simulink model "Ex_1_4_Control_Puma_2019a"  (R2019a)
settings: Solver=FixedStepAuto  StartTime=0.0  StopTime=6  FixedStep=0.01  RelTol=1e-3
libraries: simulink x6
(part 1 of 2)
settings Model: Creator=s3818101  LastModifiedBy=s3818101
settings DebuggingCC: UnconnectedInputMsg=none  UnconnectedOutputMsg=none  UnconnectedLineMsg=none
settings ModelReferenceCC: EnableRefExpFcnMdlSchedulingChecks=off
settings RTWCC: Description=Generic Real-Time Target

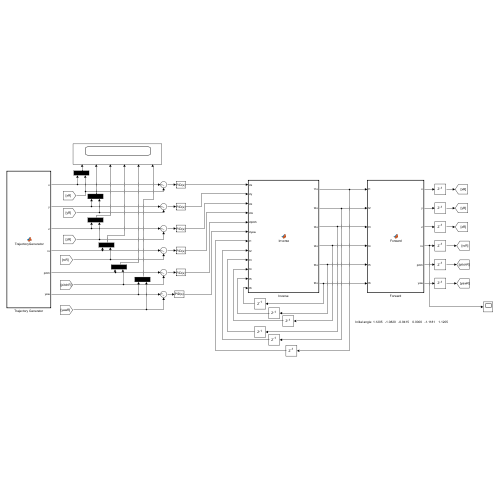
[thumbnail: Simulink's stored preview of the top-level diagram]
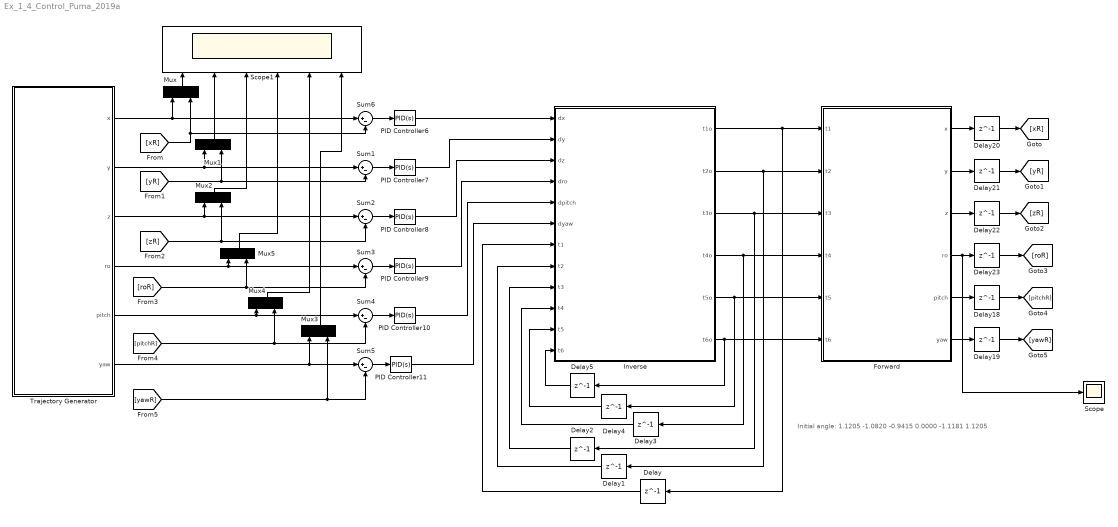
== system Ex_1_4_Control_Puma_2019a ==
  note: Initial angle: 1.1205 -1.0820 -0.9415 0.0000 -1.1181 1.1205
  Delay : Delay  DelayLength=1  InitialCondition=1.1205
  Delay1 : Delay  DelayLength=1  InitialCondition=-1.1181
  Delay18 : Delay  DelayLength=1  InitialCondition=0
  Delay19 : Delay  DelayLength=1  InitialCondition=0
  Delay2 : Delay  DelayLength=1  InitialCondition=0.001
  Delay20 : Delay  DelayLength=1  InitialCondition=0.001
  Delay21 : Delay  DelayLength=1  InitialCondition=0.001
  Delay22 : Delay  DelayLength=1  InitialCondition=0.01
  Delay23 : Delay  DelayLength=1  InitialCondition=pi
  Delay3 : Delay  DelayLength=1  InitialCondition=-0.9415
  Delay4 : Delay  DelayLength=1  InitialCondition=-1.082
  Delay5 : Delay  DelayLength=1  InitialCondition=1.1205
  "Forward " : MATLAB Function  TreatAsAtomicUnit=on
  Inverse : MATLAB Function  TreatAsAtomicUnit=on
  Mux{,1..5} (6 alike) : Mux  Inputs=2
  PID Controller10 : simulink/Continuous/PID Controller  Controller=PID  Form=Parallel  TimeDomain=Continuous-time  SampleTime=-1  IntegratorMethod=Forward Euler  ControllerParametersSource=internal  P=3.6  I=0  D=0.1  N=100  UseFilter=on  TunerSelectOption=Transfer Function Based (PID Tuner App)  InitialConditionSource=internal  InitialConditionForIntegrator=0  InitialConditionForFilter=0  DifferentiatorICPrevScaledInput=0  ExternalReset=none  TrackingMode=off  Kt=1  LimitOutput=off  UpperSaturationLimit=inf  LowerSaturationLimit=-inf  LinearizeAsGain=on  AntiWindupMode=none  Kb=1  POutMin=[]  POutMax=[]  IOutMin=[]  IOutMax=[]  DOutMin=[]  DOutMax=[]  NOutMin=[]  NOutMax=[]  SumOutMin=[]  SumOutMax=[]  SaturationOutMin=[]  SaturationOutMax=[]  PParamMin=[]  PParamMax=[]  IParamMin=[]  IParamMax=[]  DParamMin=[]  DParamMax=[]  NParamMin=[]  NParamMax=[]  KbParamMin=[]  KbParamMax=[]  KtParamMin=[]  KtParamMax=[]  KbOutMin=[]  KbOutMax=[]  KtOutMin=[]  KtOutMax=[]  IntegratorOutMin=[]  IntegratorOutMax=[]  FilterOutMin=[]  FilterOutMax=[]  SumI1OutMin=[]  SumI1OutMax=[]  SumI2OutMin=[]  SumI2OutMax=[]  SumI3OutMin=[]  SumI3OutMax=[]  SumI4OutMin=[]  SumI4OutMax=[]  SumDOutMin=[]  SumDOutMax=[]  DifferentiatorOutMin=[]  DifferentiatorOutMax=[]  FilterDiffOutCoefMin=[]  FilterDiffOutCoefMax=[]  ReciprocalOutMin=[]  ReciprocalOutMax=[]  SumDenOutMin=[]  SumDenOutMax=[]  SumNumOutMin=[]  SumNumOutMax=[]  DivideOutMin=[]  DivideOutMax=[]  IntegratorContinuousStateAttributes=''  IntegratorStateMustResolveToSignalObject=off  IntegratorRTWStateStorageClass=Auto  FilterContinuousStateAttributes=''  FilterStateMustResolveToSignalObject=off  FilterRTWStateStorageClass=Auto  ParallelPVariant=InternalParameters  IdealPVariant=Disabled  IVariant=InternalParameters  DVariant=InternalParameters  IntegratorVariant=Continuous  SatVariant=Disabled  AWVariant=Passthrough  PCopyVariant=Disabled  TRVariant=Disabled  FdbkBlocksVariant=Forward  IdealPFdbkVariant=Disabled  SatFdbkVariant=Disabled  DerivativeFilterVariant=ContFilter  NVariant=InternalParameters  NCopyVariant=Disabled  FilterICVariant=InternalICsFilter  IntegratorICVariant=InternalICs  ExternalResetVariant=Disabled  TRSumVariant=Passthrough  SumFdbkVariant=Disabled  SumVariant=Sum_PID
  PID Controller11 : simulink/Continuous/PID Controller  Controller=PID  Form=Parallel  TimeDomain=Continuous-time  SampleTime=-1  IntegratorMethod=Forward Euler  ControllerParametersSource=internal  P=3  I=0  D=0.008  N=100  UseFilter=on  TunerSelectOption=Transfer Function Based (PID Tuner App)  InitialConditionSource=internal  InitialConditionForIntegrator=0  InitialConditionForFilter=0  DifferentiatorICPrevScaledInput=0  ExternalReset=none  TrackingMode=off  Kt=1  LimitOutput=off  UpperSaturationLimit=inf  LowerSaturationLimit=-inf  LinearizeAsGain=on  AntiWindupMode=none  Kb=1  POutMin=[]  POutMax=[]  IOutMin=[]  IOutMax=[]  DOutMin=[]  DOutMax=[]  NOutMin=[]  NOutMax=[]  SumOutMin=[]  SumOutMax=[]  SaturationOutMin=[]  SaturationOutMax=[]  PParamMin=[]  PParamMax=[]  IParamMin=[]  IParamMax=[]  DParamMin=[]  DParamMax=[]  NParamMin=[]  NParamMax=[]  KbParamMin=[]  KbParamMax=[]  KtParamMin=[]  KtParamMax=[]  KbOutMin=[]  KbOutMax=[]  KtOutMin=[]  KtOutMax=[]  IntegratorOutMin=[]  IntegratorOutMax=[]  FilterOutMin=[]  FilterOutMax=[]  SumI1OutMin=[]  SumI1OutMax=[]  SumI2OutMin=[]  SumI2OutMax=[]  SumI3OutMin=[]  SumI3OutMax=[]  SumI4OutMin=[]  SumI4OutMax=[]  SumDOutMin=[]  SumDOutMax=[]  DifferentiatorOutMin=[]  DifferentiatorOutMax=[]  FilterDiffOutCoefMin=[]  FilterDiffOutCoefMax=[]  ReciprocalOutMin=[]  ReciprocalOutMax=[]  SumDenOutMin=[]  SumDenOutMax=[]  SumNumOutMin=[]  SumNumOutMax=[]  DivideOutMin=[]  DivideOutMax=[]  IntegratorContinuousStateAttributes=''  IntegratorStateMustResolveToSignalObject=off  IntegratorRTWStateStorageClass=Auto  FilterContinuousStateAttributes=''  FilterStateMustResolveToSignalObject=off  FilterRTWStateStorageClass=Auto  ParallelPVariant=InternalParameters  IdealPVariant=Disabled  IVariant=InternalParameters  DVariant=InternalParameters  IntegratorVariant=Continuous  SatVariant=Disabled  AWVariant=Passthrough  PCopyVariant=Disabled  TRVariant=Disabled  FdbkBlocksVariant=Forward  IdealPFdbkVariant=Disabled  SatFdbkVariant=Disabled  DerivativeFilterVariant=ContFilter  NVariant=InternalParameters  NCopyVariant=Disabled  FilterICVariant=InternalICsFilter  IntegratorICVariant=InternalICs  ExternalResetVariant=Disabled  TRSumVariant=Passthrough  SumFdbkVariant=Disabled  SumVariant=Sum_PID
  PID Controller6 : simulink/Continuous/PID Controller  Controller=PID  Form=Parallel  TimeDomain=Continuous-time  SampleTime=-1  IntegratorMethod=Forward Euler  ControllerParametersSource=internal  P=10  I=0  D=0  N=100  UseFilter=on  TunerSelectOption=Transfer Function Based (PID Tuner App)  InitialConditionSource=internal  InitialConditionForIntegrator=0  InitialConditionForFilter=0  DifferentiatorICPrevScaledInput=0  ExternalReset=none  TrackingMode=off  Kt=1  LimitOutput=off  UpperSaturationLimit=inf  LowerSaturationLimit=-inf  LinearizeAsGain=on  AntiWindupMode=none  Kb=1  POutMin=[]  POutMax=[]  IOutMin=[]  IOutMax=[]  DOutMin=[]  DOutMax=[]  NOutMin=[]  NOutMax=[]  SumOutMin=[]  SumOutMax=[]  SaturationOutMin=[]  SaturationOutMax=[]  PParamMin=[]  PParamMax=[]  IParamMin=[]  IParamMax=[]  DParamMin=[]  DParamMax=[]  NParamMin=[]  NParamMax=[]  KbParamMin=[]  KbParamMax=[]  KtParamMin=[]  KtParamMax=[]  KbOutMin=[]  KbOutMax=[]  KtOutMin=[]  KtOutMax=[]  IntegratorOutMin=[]  IntegratorOutMax=[]  FilterOutMin=[]  FilterOutMax=[]  SumI1OutMin=[]  SumI1OutMax=[]  SumI2OutMin=[]  SumI2OutMax=[]  SumI3OutMin=[]  SumI3OutMax=[]  SumI4OutMin=[]  SumI4OutMax=[]  SumDOutMin=[]  SumDOutMax=[]  DifferentiatorOutMin=[]  DifferentiatorOutMax=[]  FilterDiffOutCoefMin=[]  FilterDiffOutCoefMax=[]  ReciprocalOutMin=[]  ReciprocalOutMax=[]  SumDenOutMin=[]  SumDenOutMax=[]  SumNumOutMin=[]  SumNumOutMax=[]  DivideOutMin=[]  DivideOutMax=[]  IntegratorContinuousStateAttributes=''  IntegratorStateMustResolveToSignalObject=off  IntegratorRTWStateStorageClass=Auto  FilterContinuousStateAttributes=''  FilterStateMustResolveToSignalObject=off  FilterRTWStateStorageClass=Auto  ParallelPVariant=InternalParameters  IdealPVariant=Disabled  IVariant=InternalParameters  DVariant=InternalParameters  IntegratorVariant=Continuous  SatVariant=Disabled  AWVariant=Passthrough  PCopyVariant=Disabled  TRVariant=Disabled  FdbkBlocksVariant=Forward  IdealPFdbkVariant=Disabled  SatFdbkVariant=Disabled  DerivativeFilterVariant=ContFilter  NVariant=InternalParameters  NCopyVariant=Disabled  FilterICVariant=InternalICsFilter  IntegratorICVariant=InternalICs  ExternalResetVariant=Disabled  TRSumVariant=Passthrough  SumFdbkVariant=Disabled  SumVariant=Sum_PID
  PID Controller7 : simulink/Continuous/PID Controller  Controller=PID  Form=Parallel  TimeDomain=Continuous-time  SampleTime=-1  IntegratorMethod=Forward Euler  ControllerParametersSource=internal  P=6  I=0  D=0  N=100  UseFilter=on  TunerSelectOption=Transfer Function Based (PID Tuner App)  InitialConditionSource=internal  InitialConditionForIntegrator=0  InitialConditionForFilter=0  DifferentiatorICPrevScaledInput=0  ExternalReset=none  TrackingMode=off  Kt=1  LimitOutput=off  UpperSaturationLimit=inf  LowerSaturationLimit=-inf  LinearizeAsGain=on  AntiWindupMode=none  Kb=1  POutMin=[]  POutMax=[]  IOutMin=[]  IOutMax=[]  DOutMin=[]  DOutMax=[]  NOutMin=[]  NOutMax=[]  SumOutMin=[]  SumOutMax=[]  SaturationOutMin=[]  SaturationOutMax=[]  PParamMin=[]  PParamMax=[]  IParamMin=[]  IParamMax=[]  DParamMin=[]  DParamMax=[]  NParamMin=[]  NParamMax=[]  KbParamMin=[]  KbParamMax=[]  KtParamMin=[]  KtParamMax=[]  KbOutMin=[]  KbOutMax=[]  KtOutMin=[]  KtOutMax=[]  IntegratorOutMin=[]  IntegratorOutMax=[]  FilterOutMin=[]  FilterOutMax=[]  SumI1OutMin=[]  SumI1OutMax=[]  SumI2OutMin=[]  SumI2OutMax=[]  SumI3OutMin=[]  SumI3OutMax=[]  SumI4OutMin=[]  SumI4OutMax=[]  SumDOutMin=[]  SumDOutMax=[]  DifferentiatorOutMin=[]  DifferentiatorOutMax=[]  FilterDiffOutCoefMin=[]  FilterDiffOutCoefMax=[]  ReciprocalOutMin=[]  ReciprocalOutMax=[]  SumDenOutMin=[]  SumDenOutMax=[]  SumNumOutMin=[]  SumNumOutMax=[]  DivideOutMin=[]  DivideOutMax=[]  IntegratorContinuousStateAttributes=''  IntegratorStateMustResolveToSignalObject=off  IntegratorRTWStateStorageClass=Auto  FilterContinuousStateAttributes=''  FilterStateMustResolveToSignalObject=off  FilterRTWStateStorageClass=Auto  ParallelPVariant=InternalParameters  IdealPVariant=Disabled  IVariant=InternalParameters  DVariant=InternalParameters  IntegratorVariant=Continuous  SatVariant=Disabled  AWVariant=Passthrough  PCopyVariant=Disabled  TRVariant=Disabled  FdbkBlocksVariant=Forward  IdealPFdbkVariant=Disabled  SatFdbkVariant=Disabled  DerivativeFilterVariant=ContFilter  NVariant=InternalParameters  NCopyVariant=Disabled  FilterICVariant=InternalICsFilter  IntegratorICVariant=InternalICs  ExternalResetVariant=Disabled  TRSumVariant=Passthrough  SumFdbkVariant=Disabled  SumVariant=Sum_PID
  PID Controller8 : simulink/Continuous/PID Controller  Controller=PID  Form=Parallel  TimeDomain=Continuous-time  SampleTime=-1  IntegratorMethod=Forward Euler  ControllerParametersSource=internal  P=6  I=0  D=0  N=100  UseFilter=on  TunerSelectOption=Transfer Function Based (PID Tuner App)  InitialConditionSource=internal  InitialConditionForIntegrator=0  InitialConditionForFilter=0  DifferentiatorICPrevScaledInput=0  ExternalReset=none  TrackingMode=off  Kt=1  LimitOutput=off  UpperSaturationLimit=inf  LowerSaturationLimit=-inf  LinearizeAsGain=on  AntiWindupMode=none  Kb=1  POutMin=[]  POutMax=[]  IOutMin=[]  IOutMax=[]  DOutMin=[]  DOutMax=[]  NOutMin=[]  NOutMax=[]  SumOutMin=[]  SumOutMax=[]  SaturationOutMin=[]  SaturationOutMax=[]  PParamMin=[]  PParamMax=[]  IParamMin=[]  IParamMax=[]  DParamMin=[]  DParamMax=[]  NParamMin=[]  NParamMax=[]  KbParamMin=[]  KbParamMax=[]  KtParamMin=[]  KtParamMax=[]  KbOutMin=[]  KbOutMax=[]  KtOutMin=[]  KtOutMax=[]  IntegratorOutMin=[]  IntegratorOutMax=[]  FilterOutMin=[]  FilterOutMax=[]  SumI1OutMin=[]  SumI1OutMax=[]  SumI2OutMin=[]  SumI2OutMax=[]  SumI3OutMin=[]  SumI3OutMax=[]  SumI4OutMin=[]  SumI4OutMax=[]  SumDOutMin=[]  SumDOutMax=[]  DifferentiatorOutMin=[]  DifferentiatorOutMax=[]  FilterDiffOutCoefMin=[]  FilterDiffOutCoefMax=[]  ReciprocalOutMin=[]  ReciprocalOutMax=[]  SumDenOutMin=[]  SumDenOutMax=[]  SumNumOutMin=[]  SumNumOutMax=[]  DivideOutMin=[]  DivideOutMax=[]  IntegratorContinuousStateAttributes=''  IntegratorStateMustResolveToSignalObject=off  IntegratorRTWStateStorageClass=Auto  FilterContinuousStateAttributes=''  FilterStateMustResolveToSignalObject=off  FilterRTWStateStorageClass=Auto  ParallelPVariant=InternalParameters  IdealPVariant=Disabled  IVariant=InternalParameters  DVariant=InternalParameters  IntegratorVariant=Continuous  SatVariant=Disabled  AWVariant=Passthrough  PCopyVariant=Disabled  TRVariant=Disabled  FdbkBlocksVariant=Forward  IdealPFdbkVariant=Disabled  SatFdbkVariant=Disabled  DerivativeFilterVariant=ContFilter  NVariant=InternalParameters  NCopyVariant=Disabled  FilterICVariant=InternalICsFilter  IntegratorICVariant=InternalICs  ExternalResetVariant=Disabled  TRSumVariant=Passthrough  SumFdbkVariant=Disabled  SumVariant=Sum_PID
  PID Controller9 : simulink/Continuous/PID Controller  Controller=PID  Form=Parallel  TimeDomain=Continuous-time  SampleTime=-1  IntegratorMethod=Forward Euler  ControllerParametersSource=internal  P=1  I=0  D=0.01  N=100  UseFilter=on  TunerSelectOption=Transfer Function Based (PID Tuner App)  InitialConditionSource=internal  InitialConditionForIntegrator=0  InitialConditionForFilter=0  DifferentiatorICPrevScaledInput=0  ExternalReset=none  TrackingMode=off  Kt=1  LimitOutput=off  UpperSaturationLimit=inf  LowerSaturationLimit=-inf  LinearizeAsGain=on  AntiWindupMode=none  Kb=1  POutMin=[]  POutMax=[]  IOutMin=[]  IOutMax=[]  DOutMin=[]  DOutMax=[]  NOutMin=[]  NOutMax=[]  SumOutMin=[]  SumOutMax=[]  SaturationOutMin=[]  SaturationOutMax=[]  PParamMin=[]  PParamMax=[]  IParamMin=[]  IParamMax=[]  DParamMin=[]  DParamMax=[]  NParamMin=[]  NParamMax=[]  KbParamMin=[]  KbParamMax=[]  KtParamMin=[]  KtParamMax=[]  KbOutMin=[]  KbOutMax=[]  KtOutMin=[]  KtOutMax=[]  IntegratorOutMin=[]  IntegratorOutMax=[]  FilterOutMin=[]  FilterOutMax=[]  SumI1OutMin=[]  SumI1OutMax=[]  SumI2OutMin=[]  SumI2OutMax=[]  SumI3OutMin=[]  SumI3OutMax=[]  SumI4OutMin=[]  SumI4OutMax=[]  SumDOutMin=[]  SumDOutMax=[]  DifferentiatorOutMin=[]  DifferentiatorOutMax=[]  FilterDiffOutCoefMin=[]  FilterDiffOutCoefMax=[]  ReciprocalOutMin=[]  ReciprocalOutMax=[]  SumDenOutMin=[]  SumDenOutMax=[]  SumNumOutMin=[]  SumNumOutMax=[]  DivideOutMin=[]  DivideOutMax=[]  IntegratorContinuousStateAttributes=''  IntegratorStateMustResolveToSignalObject=off  IntegratorRTWStateStorageClass=Auto  FilterContinuousStateAttributes=''  FilterStateMustResolveToSignalObject=off  FilterRTWStateStorageClass=Auto  ParallelPVariant=InternalParameters  IdealPVariant=Disabled  IVariant=InternalParameters  DVariant=InternalParameters  IntegratorVariant=Continuous  SatVariant=Disabled  AWVariant=Passthrough  PCopyVariant=Disabled  TRVariant=Disabled  FdbkBlocksVariant=Forward  IdealPFdbkVariant=Disabled  SatFdbkVariant=Disabled  DerivativeFilterVariant=ContFilter  NVariant=InternalParameters  NCopyVariant=Disabled  FilterICVariant=InternalICsFilter  IntegratorICVariant=InternalICs  ExternalResetVariant=Disabled  TRSumVariant=Passthrough  SumFdbkVariant=Disabled  SumVariant=Sum_PID
  Scope : Scope
  Scope1 : Scope  NumInputPorts=6
  Sum{1..6} (6 alike) : Sum  Inputs=|+-
  Trajectory Generator : MATLAB Function  TreatAsAtomicUnit=on
  wires:
  Trajectory Generator/1(x) -> Sum6/1, Mux/1
  "Forward "/1(x) -> Delay20/1
  "Forward "/2(y) -> Delay21/1
  "Forward "/3(z) -> Delay22/1
  Inverse/1(t1o) -> Delay/1, "Forward "/1(t1)
  Inverse/2(t2o) -> Delay1/1, "Forward "/2(t2)
  Inverse/3(t3o) -> Delay2/1, "Forward "/3(t3)
  Inverse/4(t4o) -> Delay3/1, "Forward "/4(t4)
  Inverse/5(t5o) -> Delay4/1, "Forward "/5(t5)
  Inverse/6(t6o) -> Delay5/1, "Forward "/6(t6)
  PID Controller6/1 -> Inverse/1(dx)
  PID Controller7/1 -> Inverse/2(dy)
  PID Controller8/1 -> Inverse/3(dz)
  PID Controller9/1 -> Inverse/4(dro)
  PID Controller10/1 -> Inverse/5(dpitch)
  PID Controller11/1 -> Inverse/6(dyaw)
  Delay/1 -> Inverse/7(t1)
  Delay1/1 -> Inverse/8(t2)
  Delay2/1 -> Inverse/9(t3)
  Delay3/1 -> Inverse/10(t4)
  Delay4/1 -> Inverse/11(t5)
  Delay5/1 -> Inverse/12(t6)
  Delay20/1 -> [xR]
  Delay21/1 -> [yR]
  Delay22/1 -> [zR]
  "Forward "/4(ro) -> Delay23/1, Scope/1
  "Forward "/5(pitch) -> Delay18/1
  "Forward "/6(yaw) -> Delay19/1
  Sum6/1 -> PID Controller6/1
  Trajectory Generator/2(y) -> Sum1/1, Mux1/1
  Sum1/1 -> PID Controller7/1
  [xR] -> Sum6/2, Mux/2
  [yR] -> Sum1/2, Mux1/2
  Sum2/1 -> PID Controller8/1
  Trajectory Generator/3(z) -> Sum2/1, Mux2/1
  [zR] -> Sum2/2, Mux2/2
  Trajectory Generator/4(ro) -> Sum3/1, Mux5/1
  Sum3/1 -> PID Controller9/1
  [roR] -> Sum3/2, Mux5/2
  Trajectory Generator/5(pitch) -> Sum4/1, Mux4/1
  Sum4/1 -> PID Controller10/1
  [pitchR] -> Sum4/2, Mux4/2
  Trajectory Generator/6(yaw) -> Sum5/1, Mux3/1
  [yawR] -> Sum5/2, Mux3/2
  Sum5/1 -> PID Controller11/1
  Mux/1 -> Scope1/1
  Mux1/1 -> Scope1/2
  Mux2/1 -> Scope1/3
  Mux5/1 -> Scope1/4
  Mux4/1 -> Scope1/5
  Mux3/1 -> Scope1/6
  Delay18/1 -> [pitchR]
  Delay19/1 -> [yawR]
  Delay23/1 -> [roR]

== matlab function Ex_1_4_Control_Puma_2019a/Forward  ==
  data: x output; y output; t1 input; t2 input; t3 input; t4 input; t5 input; t6 input; z output; ro output; pitch output; yaw output
function [x, y, z, ro, pitch, yaw] = Forward(t1, t2, t3, t4, t5, t6)


Tf_matrix = [
  sin(t6)*(cos(t4)*sin(t1) + sin(t4)*(cos(t1)*sin(t2)*sin(t3) - cos(t1)*cos(t2)*cos(t3))) + cos(t6)*(cos(t5)*(sin(t1)*sin(t4) - cos(t4)*(cos(t1)*sin(t2)*sin(t3) - cos(t1)*cos(t2)*cos(t3))) - sin(t5)*(cos(t1)*cos(t2)*sin(t3) + cos(t1)*cos(t3)*sin(t2))), cos(t6)*(cos(t4)*sin(t1) + sin(t4)*(cos(t1)*sin(t2)*sin(t3) - cos(t1)*cos(t2)*cos(t3))) - sin(t6)*(cos(t5)*(sin(t1)*sin(t4) - cos(t4)*(cos(t1)*sin(t2)*sin(t3) - cos(t1)*cos(t2)*cos(t3))) - sin(t5)*(cos(t1)*cos(t2)*sin(t3) + cos(t1)*cos(t3)*sin(t2))), - sin(t5)*(sin(t1)*sin(t4) - cos(t4)*(cos(t1)*sin(t2)*sin(t3) - cos(t1)*cos(t2)*cos(t3))) - cos(t5)*(cos(t1)*cos(t2)*sin(t3) + cos(t1)*cos(t3)*sin(t2)), (2159*cos(t1)*cos(t2))/5000 - (3*sin(t1))/20 - (sin(t5)*(sin(t1)*sin(t4) - cos(t4)*(cos(t1)*sin(t2)*sin(t3) - cos(t1)*cos(t2)*cos(t3))))/10 - (cos(t5)*(cos(t1)*cos(t2)*sin(t3) + cos(t1)*cos(t3)*sin(t2)))/10 - (203*cos(t1)*sin(t2)*sin(t3))/10000 + (203*cos(t1)*cos(t2)*cos(t3))/10000 - (2159*cos(t1)*cos(t2)*sin(t3))/5000 - (2159*cos(t1)*cos(t3)*sin(t2))/5000;
- sin(t6)*(cos(t1)*cos(t4) - sin(t4)*(sin(t1)*sin(t2)*sin(t3) - cos(t2)*cos(t3)*sin(t1))) - cos(t6)*(cos(t5)*(cos(t1)*sin(t4) + cos(t4)*(sin(t1)*sin(t2)*sin(t3) - cos(t2)*cos(t3)*sin(t1))) + sin(t5)*(cos(t2)*sin(t1)*sin(t3) + cos(t3)*sin(t1)*sin(t2))), sin(t6)*(cos(t5)*(cos(t1)*sin(t4) + cos(t4)*(sin(t1)*sin(t2)*sin(t3) - cos(t2)*cos(t3)*sin(t1))) + sin(t5)*(cos(t2)*sin(t1)*sin(t3) + cos(t3)*sin(t1)*sin(t2))) - cos(t6)*(cos(t1)*cos(t4) - sin(t4)*(sin(t1)*sin(t2)*sin(t3) - cos(t2)*cos(t3)*sin(t1))),   sin(t5)*(cos(t1)*sin(t4) + cos(t4)*(sin(t1)*sin(t2)*sin(t3) - cos(t2)*cos(t3)*sin(t1))) - cos(t5)*(cos(t2)*sin(t1)*sin(t3) + cos(t3)*sin(t1)*sin(t2)), (3*cos(t1))/20 + (2159*cos(t2)*sin(t1))/5000 + (sin(t5)*(cos(t1)*sin(t4) + cos(t4)*(sin(t1)*sin(t2)*sin(t3) - cos(t2)*cos(t3)*sin(t1))))/10 - (cos(t5)*(cos(t2)*sin(t1)*sin(t3) + cos(t3)*sin(t1)*sin(t2)))/10 - (2159*cos(t2)*sin(t1)*sin(t3))/5000 - (2159*cos(t3)*sin(t1)*sin(t2))/5000 - (203*sin(t1)*sin(t2)*sin(t3))/10000 + (203*cos(t2)*cos(t3)*sin(t1))/10000;
                                                                                          sin(t4)*sin(t6)*(cos(t2)*sin(t3) + cos(t3)*sin(t2)) - cos(t6)*(sin(t5)*(cos(t2)*cos(t3) - sin(t2)*sin(t3)) + cos(t4)*cos(t5)*(cos(t2)*sin(t3) + cos(t3)*sin(t2))),                                                                                         sin(t6)*(sin(t5)*(cos(t2)*cos(t3) - sin(t2)*sin(t3)) + cos(t4)*cos(t5)*(cos(t2)*sin(t3) + cos(t3)*sin(t2))) + cos(t6)*sin(t4)*(cos(t2)*sin(t3) + cos(t3)*sin(t2)),                                                       cos(t4)*sin(t5)*(cos(t2)*sin(t3) + cos(t3)*sin(t2)) - cos(t5)*(cos(t2)*cos(t3) - sin(t2)*sin(t3)),                                                                                                              (2159*sin(t2)*sin(t3))/5000 - (2159*cos(t2)*cos(t3))/5000 - (203*cos(t2)*sin(t3))/10000 - (203*cos(t3)*sin(t2))/10000 - (2159*sin(t2))/5000 - (cos(t5)*(cos(t2)*cos(t3) - sin(t2)*sin(t3)))/10 + (cos(t4)*sin(t5)*(cos(t2)*sin(t3) + cos(t3)*sin(t2)))/10;
                                                                                                                                                                                                                                                          0,                                                                                                                                                                                                                                                         0,                                                                                                                                                       0,                                                                                                                                                                                                                                                                                                                                                                      1;];


E = Tf_matrix;
x = E(1, 4);
y = E(2, 4);
z = E(3, 4);

res = rotm2eul(E(1:3, 1:3), "XYZ");

ro = res(1);
if ro <= 0
    ro = ro + pi - 0.001;
% elseif

end
pitch = res(2);
yaw = res(3);
% if yaw < 0 
%     yaw = yaw + pi;
% end


% pitch = asin(-E(3,1));
% ro = atan2(E(2,1)/cos(pitch), E(1,1)/cos(pitch));
% if ro < 0 
%     ro = ro + pi;
% end
% yaw = atan2(E(3,2)/cos(pitch), E(3,3)/cos(pitch));
% 
% ro = atan2(Tf_matrix(3, 2), Tf_matrix(3, 3));
% 
% pitch = atan2(-Tf_matrix(3, 1), sqrt(Tf_matrix(3, 2)^2 + Tf_matrix(3, 3)^2));
% 
% yaw = atan2(Tf_matrix(2, 1), Tf_matrix(1, 1));
% 
% if ro < 0
%     ro = ro + pi;
% end
% if pitch < 0
%     pitch = pitch + pi;
% end
% if yaw < 0
%     yaw = yaw + pi;
% end

== matlab function Ex_1_4_Control_Puma_2019a/Trajectory Generator ==
  data: x output; y output; z output; ro output; pitch output; yaw output
function [x,y,z, ro, pitch, yaw] = TrajectoryGenerator

persistent i starttime

traj = [0.0240000000000000     0.126000000000000       0;];
for j = 1:71
    traj = [traj;0.0240000000000000     0.126000000000000       0];
end

traj = [ traj;
0.0240000000000000     0.126000000000000       0;
0.0240000000000000     0.126000000000000       0;
0.0240000000000000     0.126000000000000       0;
0.0240000000000000     0.126000000000000       0;
0.0240000000000000     0.126000000000000       0;
0.0240000000000000      0.126000000000000       0;
0.0240000000000000      0.126000000000000       0;
0.0240000000000000      0.126000000000000       0;
0.0240000000000000      0.126000000000000       0;
0.0240000000000000      0.126000000000000       0;
0.0240000000000000      0.126000000000000       0;
0.0240000000000000      0.126000000000000       0;
0.0240000000000000      0.126000000000000       0;
0.0240000000000000      0.126000000000000       0;
0.0240000000000000      0.126000000000000       0;
0.0240000000000000      0.126000000000000       0;
0.0240000000000000      0.126000000000000       0;
0.0240000000000000      0.126000000000000       0;
0.0240000000000000      0.126000000000000       0;
0.0240000000000000      0.125947956521739       0;
0.0240000000000000      0.125605565217391       0;
0.0240000000000000      0.124742739130435       0;
0.0240000000000000      0.123195130434783       0;
0.0240000000000000      0.120864130434783       0;
0.0240000000000000      0.117716869565217       0;
0.0240000000000000      0.113786217391304       0;
0.0240000000000000      0.109170782608696       0;
0.0240000000000000      0.104034913043478       0;
0.0240000000000000      0.0986086956521739      0;
0.0240000000000000      0.0931304347826087      0;
0.0240000000000000      0.0876521739130435      0;
0.0240000000000000      0.0821739130434783      0;
0.0240000000000000      0.0766956521739131      0;
0.0240000000000000      0.0712173913043478      0;
0.0240000000000000      0.0657391304347826      0;
0.0240000000000000      0.0602608695652174      0;
0.0240000000000000      0.0547826086956522      0;
0.0240000000000000      0.0493043478260870      0;
0.0240000000000000      0.0438260869565218      0;
0.0240000000000000      0.0383478260869565      0;
0.0240000000000000      0.0328695652173913      0;
0.0240000000000000      0.0273913043478261      0;
0.0240000000000000      0.0219650869565218      4.75000000000000e-05;
0.0240000000000000      0.0168292173913044      0.000360000000000000;
0.0240000000000000      0.0122137826086957      0.00114750000000000;
0.0240000000000000      0.00828313043478262     0.00256000000000000;
0.0240000000000000      0.00513586956521740     0.00468750000000000;
0.0240000000000000      0.00280486956521740     0.00756000000000000;
0.0240000000000000      0.00125726086956523     0.0111475000000000;
0.0240000000000000      0.000394434782608713    0.0153600000000000;
0.0240000000000000      5.20434782608926e-05    0.0200475000000000;
0.0240000000000000      3.12250225675825e-17    0.0250000000000000;
0.0240000000000000      0       0.0300000000000000;
0.0240000000000000      0       0.0350000000000000;
0.0240000000000000      0       0.0400000000000000;
0.0240000000000000      0       0.0450000000000000;
0.0240000000000000      0       0.0500000000000000;
0.0240000000000000      0       0.0550000000000000;
0.0240000000000000      0       0.0600000000000000;
0.0240000000000000      0       0.0650000000000000;
0.0240000000000000      0       0.0700000000000000;
0.0240000000000000      0       0.0750000000000000;
0.0240346956521739      5.20434782608695e-05    0.0799111956521739;
0.0242629565217391      0.000394434782608696    0.0843269565217391;
0.0248381739130435      0.00125726086956522     0.0878546739130435;
0.0258699130434783      0.00280486956521739     0.0902139130434783;
0.0274239130434783      0.00513586956521739     0.0912364130434783;
0.0295220869565217      0.00828313043478261     0.0908660869565217;
0.0321425217391304      0.0122137826086957      0.0891590217391304;
0.0352194782608696      0.0168292173913044      0.0862834782608696;
0.0386433913043478      0.0219650869565218      0.0825198913043478;
0.0422608695652174      0.0273913043478261      0.0782608695652174;
0.0459130434782609      0.0328695652173913      0.0739130434782609;
0.0495652173913043      0.0383478260869565      0.0695652173913044;
0.0532173913043478      0.0438260869565217      0.0652173913043478;
0.0568695652173913      0.0493043478260870      0.0608695652173913;
0.0605217391304348      0.0547826086956522      0.0565217391304348;
0.0641739130434783      0.0602608695652174      0.0521739130434783;
0.0678260869565217      0.0657391304347826      0.0478260869565217;
0.0714782608695652      0.0712173913043478      0.0434782608695652;
0.0751304347826087      0.0766956521739131      0.0391304347826087;
0.0787826086956522      0.0821739130434783      0.0347826086956522;
0.0824347826086957      0.0876521739130435      0.0304347826086957;
0.0860869565217391      0.0931304347826087      0.0260869565217391;
0.0897391304347826      0.0986086956521739      0.0217391304347826;
0.0933566086956522      0.103982869565217       0.0174326086956522;
0.0967805217391304      0.108776347826087       0.0133565217391304;
0.0998574782608696      0.112528956521739       0.00969347826086957;
0.102477913043478       0.114912000000000       0.00657391304347827;
0.104576086956522       0.115728260869565       0.00407608695652174;
0.106130086956522       0.114912000000000       0.00222608695652175;
0.107161826086957       0.112528956521739       0.000997826086956527;
0.107737043478261       0.108776347826087       0.000313043478260878;
0.107965304347826       0.103982869565217       4.13043478261002e-05;
0.108000000000000       0.0986086956521739      2.42861286636753e-17;
0.108000000000000       0.0931304347826087      0;
0.108000000000000       0.0876521739130435      0;
0.108000000000000       0.0821739130434783      0;
0.108000000000000       0.0766956521739131      0;
0.108000000000000       0.0712173913043478      0;
0.108000000000000       0.0657391304347826      0;
0.108000000000000       0.0602608695652174      0;
0.108000000000000       0.0547826086956522      0;
0.108000000000000       0.0493043478260870      0;
0.108000000000000       0.0438260869565218      0;
0.108000000000000       0.0383478260869565      0;
0.108000000000000       0.0328695652173913      0;
0.108000000000000       0.0273913043478261      0;
0.108000000000000       0.0219650869565218      4.75000000000000e-05;
0.108000000000000       0.0168292173913044      0.000360000000000000;
0.108000000000000       0.0122137826086957      0.00114750000000000;
0.108000000000000       0.00828313043478262     0.00256000000000000;
0.108000000000000       0.00513586956521740     0.00468750000000000;
0.108000000000000       0.00280486956521740     0.00756000000000000;
0.108000000000000       0.00125726086956523     0.0111475000000000;
0.108000000000000       0.000394434782608713    0.0153600000000000;
0.108000000000000       5.20434782608926e-05    0.0200475000000000;
0.108000000000000       3.12250225675825e-17    0.0250000000000000;
0.108000000000000       0       0.0300000000000000;
0.108000000000000       0       0.0350000000000000;
0.108000000000000       0       0.0400000000000000;
0.108000000000000       0       0.0450000000000000;
0.108000000000000       0       0.0500000000000000;
0.108000000000000       0       0.0550000000000000;
0.108000000000000       0       0.0600000000000000;
0.108000000000000       0       0.0650000000000000;
0.108000000000000       0       0.0700000000000000;
0.108000000000000       0       0.0750000000000000;
0.107960100000000       3.13500000000000e-05    0.0799050000000000;
0.107697600000000       0.000237600000000000    0.0842800000000000;
0.107036100000000       0.000757350000000000    0.0877050000000000;
0.105849600000000       0.00168960000000000     0.0898800000000000;
0.104062500000000       0.00309375000000000     0.0906250000000000;
0.101649600000000       0.00498960000000000     0.0898800000000000;
0.0986361000000000      0.00735735000000001     0.0877050000000000;
0.0950976000000000      0.0101376000000000      0.0842800000000000;
0.0911601000000000      0.0132313500000000      0.0799050000000000;
0.0869999999999999      0.0165000000000000      0.0750000000000000;
0.0828000000000000      0.0198000000000000      0.0700000000000000;
0.0786000000000000      0.0231000000000000      0.0650000000000000;
0.0744000000000000      0.0264000000000000      0.0600000000000000;
0.0702000000000000      0.0297000000000000      0.0550000000000000;
0.0660000000000000      0.0330000000000000      0.0500000000000000;
0.0618000000000000      0.0363000000000000      0.0450000000000000;
0.0576000000000000      0.0396000000000000      0.0400000000000000;
0.0534000000000000      0.0429000000000000      0.0350000000000000;
0.0492000000000000      0.0462000000000000      0.0300000000000000;
0.0450000000000000      0.0495000000000000      0.0250000000000000;
0.0408798000000000      0.0527686500000000      0.0200475000000000;
0.0372048000000000      0.0558624000000000      0.0153600000000000;
0.0343278000000000      0.0586426500000000      0.0111475000000000;
0.0325008000000000      0.0610104000000000      0.00756000000000001;
0.0318750000000000      0.0629062500000000      0.00468750000000001;
0.0325008000000000      0.0643104000000000      0.00256000000000001;
0.0343278000000000      0.0652426500000000      0.00114750000000001;
0.0372048000000000      0.0657624000000000      0.000360000000000018;
0.0408798000000000      0.0659686500000000      4.75000000000180e-05;
0.0450000000000000      0.0660000000000000      3.12250225675825e-17;
0.0492000000000000      0.0660000000000000      0;
0.0534000000000000      0.0660000000000000      0;
0.0576000000000000      0.0660000000000000      0;
0.0618000000000000      0.0660000000000000      0;
0.0660000000000000      0.0660000000000000      0;
0.0702000000000000      0.0660000000000000      0;
0.0744000000000000      0.0660000000000000      0;
0.0786000000000000      0.0660000000000000      0;
0.0828000000000000      0.0660000000000000      0;
0.0870000000000000      0.0660000000000000      0;
0.0911601000000000      0.0660000000000000      4.75000000000000e-05;
0.0950976000000000      0.0660000000000000      0.000360000000000000;
0.0986361000000000      0.0660000000000000      0.00114750000000000;
0.101649600000000       0.0660000000000000      0.00256000000000000;
0.104062500000000       0.0660000000000000      0.00468750000000000;
0.105849600000000       0.0660000000000000      0.00756000000000000;
0.107036100000000       0.0660000000000000      0.0111475000000000;
0.107697600000000       0.0660000000000000      0.0153600000000000;
0.107960100000000       0.0660000000000000      0.0200475000000000;
0.108000000000000       0.0660000000000000      0.0250000000000000;
0.108000000000000       0.0660000000000000      0.0300000000000000;
0.108000000000000       0.0660000000000000      0.0350000000000000;
0.108000000000000       0.0660000000000000      0.0400000000000000;
0.108000000000000       0.0660000000000000      0.0450000000000000;
0.108000000000000       0.0660000000000000      0.0500000000000000;
0.108000000000000       0.0660000000000000      0.0550000000000000;
0.108000000000000       0.0660000000000000      0.0600000000000000;
0.108000000000000       0.0660000000000000      0.0650000000000000;
0.108000000000000       0.0660000000000000      0.0700000000000000;
0.108000000000000       0.0660000000000000      0.0750000000000000;
0.108007600000000       0.0660285000000000      0.0799050000000000;
0.108057600000000       0.0662160000000000      0.0842800000000000;
0.108183600000000       0.0666885000000000      0.0877050000000000;
0.108409600000000       0.0675360000000000      0.0898800000000000;
0.108750000000000       0.0688125000000000      0.0906250000000000;
0.109209600000000       0.0705360000000000      0.0898800000000000;
0.109783600000000       0.0726885000000000      0.0877050000000000;
0.110457600000000       0.0752160000000000      0.0842800000000000;
0.111207600000000       0.0780285000000000      0.0799050000000000;
0.112000000000000       0.0810000000000000      0.0750000000000000;
0.112800000000000       0.0840000000000000      0.0700000000000000;
0.113600000000000       0.0870000000000000      0.0650000000000000;
0.114400000000000       0.0900000000000000      0.0600000000000000;
0.115200000000000       0.0930000000000000      0.0550000000000000;
0.116000000000000       0.0960000000000000      0.0500000000000000;
0.116800000000000       0.0990000000000000      0.0450000000000000;
0.117600000000000       0.102000000000000       0.0400000000000000;
0.118400000000000       0.105000000000000       0.0350000000000000;
0.119200000000000       0.108000000000000       0.0300000000000000;
0.120000000000000       0.111000000000000       0.0250000000000000;
0.120792400000000       0.113971500000000       0.0200475000000000;
0.121542400000000       0.116784000000000       0.0153600000000000;
0.122216400000000       0.119311500000000       0.0111475000000000;
0.122790400000000       0.121464000000000       0.00756000000000001;
0.123250000000000       0.123187500000000       0.00468750000000001;
0.123590400000000       0.124464000000000       0.00256000000000001;
0.123816400000000       0.125311500000000       0.00114750000000001;
0.123942400000000       0.125784000000000       0.000360000000000018;
0.123992400000000       0.125971500000000       4.75000000000180e-05;
0.124000000000000       0.126000000000000       3.12250225675825e-17;
0.124000000000000       0.126000000000000       0;
0.124000000000000       0.126000000000000       0;
0.124000000000000       0.126000000000000       0;
0.124000000000000       0.126000000000000       0;
0.124000000000000       0.126000000000000       0;
0.124000000000000       0.126000000000000       0;
0.124000000000000       0.126000000000000       0;
0.124000000000000       0.126000000000000       0;
0.124000000000000       0.126000000000000       0;
0.124000000000000       0.126000000000000       0;
0.124000000000000       0.125947956521739       0;
0.124000000000000       0.125605565217391       0;
0.124000000000000       0.124742739130435       0;
0.124000000000000       0.123195130434783       0;
0.124000000000000       0.120864130434783       0;
0.124000000000000       0.117716869565217       0;
0.124000000000000       0.113786217391304       0;
0.124000000000000       0.109170782608696       0;
0.124000000000000       0.104034913043478       0;
0.124000000000000       0.0986086956521739      0;
0.124000000000000       0.0931304347826087      0;
0.124000000000000       0.0876521739130435      0;
0.124000000000000       0.0821739130434783      0;
0.124000000000000       0.0766956521739131      0;
0.124000000000000       0.0712173913043478      0;
0.124000000000000       0.0657391304347826      0;
0.124000000000000       0.0602608695652174      0;
0.124000000000000       0.0547826086956522      0;
0.124000000000000       0.0493043478260870      0;
0.124000000000000       0.0438260869565218      0;
0.124000000000000       0.0383478260869565      0;
0.124000000000000       0.0328695652173913      0;
0.124000000000000       0.0273913043478261      0;
0.124000000000000       0.0219650869565218      4.75000000000000e-05;
0.124000000000000       0.0168292173913044      0.000360000000000000;
0.124000000000000       0.0122137826086957      0.00114750000000000;
0.124000000000000       0.00828313043478262     0.00256000000000000;
0.124000000000000       0.00513586956521740     0.00468750000000000;
0.124000000000000       0.00280486956521740     0.00756000000000000;
0.124000000000000       0.00125726086956523     0.0111475000000000;
0.124000000000000       0.000394434782608713    0.0153600000000000;
0.124000000000000       5.20434782608926e-05    0.0200475000000000;
0.124000000000000       3.12250225675825e-17    0.0250000000000000;
0.124000000000000       0       0.0300000000000000;
0.124000000000000       0       0.0350000000000000;
0.124000000000000       0       0.0400000000000000;
0.124000000000000       0       0.0450000000000000;
0.124000000000000       0       0.0500000000000000;
0.124000000000000       0       0.0550000000000000;
0.124000000000000       0       0.0600000000000000;
0.124000000000000       0       0.0650000000000000;
0.124000000000000       0       0.0700000000000000;
0.124000000000000       0       0.0750000000000000;
0.124034695652174       5.20434782608695e-05    0.0799111956521739;
0.124262956521739       0.000394434782608696    0.0843269565217391;
0.124838173913043       0.00125726086956522     0.0878546739130435;
0.125869913043478       0.00280486956521739     0.0902139130434783;
0.127423913043478       0.00513586956521739     0.0912364130434783;
0.129522086956522       0.00828313043478261     0.0908660869565217;
0.132142521739130       0.0122137826086957      0.0891590217391304;
0.135219478260870       0.0168292173913044      0.0862834782608696;
0.138643391304348       0.0219650869565218      0.0825198913043478;
0.142260869565217       0.0273913043478261      0.0782608695652174;
0.145913043478261       0.0328695652173913      0.0739130434782609;
0.149565217391304       0.0383478260869565      0.0695652173913044;
0.153217391304348       0.0438260869565217      0.0652173913043478;
0.156869565217391       0.0493043478260870      0.0608695652173913;
0.160521739130435       0.0547826086956522      0.0565217391304348;
0.164173913043478       0.0602608695652174      0.0521739130434783;
0.167826086956522       0.0657391304347826      0.0478260869565217;
0.171478260869565       0.0712173913043478      0.0434782608695652;
0.175130434782609       0.0766956521739131      0.0391304347826087;
0.178782608695652       0.0821739130434783      0.0347826086956522;
0.182434782608696       0.0876521739130435      0.0304347826086957;
0.186086956521739       0.0931304347826087      0.0260869565217391;
0.189739130434783       0.0986086956521739      0.0217391304347826;
0.193356608695652       0.103982869565217       0.0174326086956522;
0.196780521739130       0.108776347826087       0.0133565217391304;
0.199857478260870       0.112528956521739       0.00969347826086957;
0.202477913043478       0.114912000000000       0.00657391304347827;
0.204576086956522       0.115728260869565       0.00407608695652174;
0.206130086956522       0.114912000000000       0.00222608695652175;
0.207161826086957       0.112528956521739       0.000997826086956527;
0.207737043478261       0.108776347826087       0.000313043478260878;
0.207965304347826       0.103982869565217       4.13043478261002e-05;
0.208000000000000       0.0986086956521739      2.42861286636753e-17;
0.208000000000000       0.0931304347826087      0;
0.208000000000000       0.0876521739130435      0;
0.208000000000000       0.0821739130434783      0;
0.208000000000000       0.0766956521739131      0;
0.208000000000000       0.0712173913043478      0;
0.208000000000000       0.0657391304347826      0;
0.208000000000000       0.0602608695652174      0;
0.208000000000000       0.0547826086956522      0;
0.208000000000000       0.0493043478260870      0;
0.208000000000000       0.0438260869565218      0;
0.208000000000000       0.0383478260869565      0;
0.208000000000000       0.0328695652173913      0;
0.208000000000000       0.0273913043478261      0;
0.208000000000000       0.0219650869565218      4.75000000000000e-05;
0.208000000000000       0.0168292173913044      0.000360000000000000;
0.208000000000000       0.0122137826086957      0.00114750000000000;
0.208000000000000       0.00828313043478262     0.00256000000000000;
0.208000000000000       0.00513586956521740     0.00468750000000000;
0.208000000000000       0.00280486956521740     0.00756000000000000;
0.208000000000000       0.00125726086956523     0.0111475000000000;
0.208000000000000       0.000394434782608713    0.0153600000000000;
0.208000000000000       5.20434782608926e-05    0.0200475000000000;
0.208000000000000       3.12250225675825e-17    0.0250000000000000;
0.208000000000000       0       0.0300000000000000;
0.208000000000000       0       0.0350000000000000;
0.208000000000000       0       0.0400000000000000;
0.208000000000000       0       0.0450000000000000;
0.208000000000000       0       0.0500000000000000;
0.208000000000000       0       0.0550000000000000;
0.208000000000000       0       0.0600000000000000;
0.208000000000000       0       0.0650000000000000;
0.208000000000000       0       0.0700000000000000;
0.208000000000000       0       0.0750000000000000;
0.207960100000000       3.13500000000000e-05    0.0799050000000000;
0.207697600000000       0.000237600000000000    0.0842800000000000;
0.207036100000000       0.000757350000000000    0.0877050000000000;
0.205849600000000       0.00168960000000000     0.0898800000000000;
0.204062500000000       0.00309375000000000     0.0906250000000000;
0.201649600000000       0.00498960000000000     0.0898800000000000;
0.198636100000000       0.00735735000000001     0.0877050000000000;
0.195097600000000       0.0101376000000000      0.0842800000000000;
0.191160100000000       0.0132313500000000      0.0799050000000000;
0.187000000000000       0.0165000000000000      0.0750000000000000;
0.182800000000000       0.0198000000000000      0.0700000000000000;
0.178600000000000       0.0231000000000000      0.0650000000000000;
0.174400000000000       0.0264000000000000      0.0600000000000000;
0.170200000000000       0.0297000000000000      0.0550000000000000;
0.166000000000000       0.0330000000000000      0.0500000000000000;
0.161800000000000       0.0363000000000000      0.0450000000000000;
0.157600000000000       0.0396000000000000      0.0400000000000000;
0.153400000000000       0.0429000000000000      0.0350000000000000;
0.149200000000000       0.0462000000000000      0.0300000000000000;
0.145000000000000       0.0495000000000000      0.0250000000000000;
0.140879800000000       0.0527686500000000      0.0200475000000000;
0.137204800000000       0.0558624000000000      0.0153600000000000;
0.134327800000000       0.0586426500000000      0.0111475000000000;
0.132500800000000       0.0610104000000000      0.00756000000000001;
0.131875000000000       0.0629062500000000      0.00468750000000001;
0.132500800000000       0.0643104000000000      0.00256000000000001;
0.134327800000000       0.0652426500000000      0.00114750000000001;
0.137204800000000       0.0657624000000000      0.000360000000000018;
0.140879800000000       0.0659686500000000      4.75000000000180e-05;
0.145000000000000       0.0660000000000000      3.12250225675825e-17;
0.149200000000000       0.0660000000000000      0;
0.153400000000000       0.0660000000000000      0;
0.157600000000000       0.0660000000000000      0;
0.161800000000000       0.0660000000000000      0;
0.166000000000000       0.0660000000000000      0;
0.170200000000000       0.0660000000000000      0;
0.174400000000000       0.0660000000000000      0;
0.178600000000000       0.0660000000000000      0;
0.182800000000000       0.0660000000000000      0;
0.187000000000000       0.0660000000000000      0;
0.191656960000000       0.0660000000000000      0;
0.197657920000000       0.0660000000000000      0;
0.203591680000000       0.0660000000000000      0;
0.207240640000000       0.0660000000000000      0;
0.208000000000000       0.0660000000000000      0];

offset = 0.25;
traj(:, 1:2) = traj(:, 1:2) + offset;

if isempty(i)
    i = 1;
end

x = traj(i,1);
y = traj(i,2);
z = traj(i,3);
ro = pi - 0.01;
pitch = 0;
yaw = 0;

if i < length(traj)
    i = i + 1;
end
